simulink model "MultipleAccessTechniques"  (R2019a)
settings: Solver=VariableStepAuto  StartTime=0.0  StopTime=10  RelTol=1e-3
libraries: commdigbbndpm3 x2, commchan3 x1, commrandsrc3 x1, commsink2 x1, commfilt2 x1, commseqgen3 x1, commutil2 x1
settings Model: Creator=se305  LastModifiedBy=se305

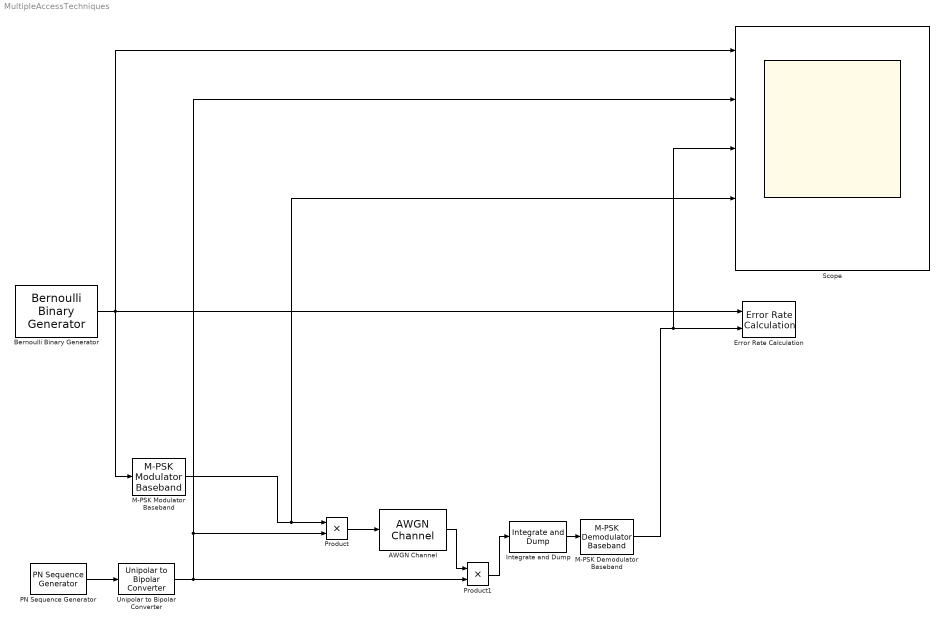
== system MultipleAccessTechniques ==
  AWGN Channel : commchan3/AWGN Channel  InputProcessing=Columns as channels (frame based)  seed=67  noiseMode="Signal to noise ratio  (Eb/No)"  EbNodB=EbNo  EsNodB=10  SNRdB=10  bitsPerSym=1  Ps=1  Tsym=1*(0.001/15)  variance=1
      settings: SourceProductName=Communications Toolbox
  Bernoulli Binary Generator : commrandsrc3/Bernoulli Binary Generator  ProbabilityOfZero=0.5  SeedSource=Auto  Seed=0  SampleTime=0.001  SamplesPerFrame=1  OutputDataType=double  SimulateUsing=Interpreted execution
      settings: SourceProductName=Communications Toolbox
  Error Rate Calculation : commsink2/Error Rate Calculation  N=0  st_delay=0  cp_mode=Entire frame  subframe=[]  PMode=Workspace  WsName=ErrorVec  RsMode2=off  stop=off  numErr=100  maxBits=1e6
      settings: SourceProductName=Communications Toolbox
  Integrate and Dump : commfilt2/Integrate and Dump  obssamples=15  offsetsamples=0  nodump=on  roundingMode=Floor  overflowMode=off  outputDataTypeStr=Inherit: Same as accumulator  outputLastDataTypeStr=Inherit: Same as accumulator
      settings: SourceProductName=Communications Toolbox
  M-PSK Demodulator Baseband : commdigbbndpm3/M-PSK Demodulator Baseband  M=2  OutType=Bit  DecType=Hard decision  VarSource=Dialog  Variance=1  Dec=Binary  Mapping=[0:7]  Ph=0  outDtype1=Inherit via internal rule  outDtype2=Inherit via internal rule  derotateFactorWordLen=16  derotateFactorDataTypeStr=Inherit: Same word length as input  derotateFactorLastDataTypeStr=Inherit: Same word length as input
      settings: SourceProductName=Communications Toolbox
  M-PSK Modulator Baseband : commdigbbndpm3/M-PSK Modulator Baseband  M=2  InType=Bit  Enc=Binary  Mapping=[0:7]  Ph=0  outDtype=double  outWordLen=16  outUDDataType=sfix(16)  outFracLenMode=Best precision  outFracLen=15  outDataTypeStr=double  outLastDataTypeStr=double
      settings: SourceProductName=Communications Toolbox
  PN Sequence Generator : commseqgen3/PN Sequence Generator  poly=[4 3 0]  ini_sta=[0 0 0 1]  outBitMaskSource=Dialog parameter  shift=0  outVarSiz=off  maxOutSizeMode=Dialog parameter  maxOutSize=[10 1]  Ts=0.001/15  sampPerFrame=1  reset=off  bitPackedOutputs=off  outDataType=double  numPackedBits=8  bitPackDataSigned=off  bitPackedOutDType=double
      settings: SourceProductName=Communications Toolbox
  Product : Product
  Product1 : Product
  Scope : Scope  NumInputPorts=5
  Unipolar to Bipolar Converter : commutil2/Unipolar to Bipolar Converter  M=2  polarity=Positive  dataType=Inherit via internal rule
      settings: SourceProductName=Communications Toolbox
  wires:
  M-PSK Demodulator Baseband/1 -> Scope/3, Error Rate Calculation/2
  AWGN Channel/1 -> Product1/1
  PN Sequence Generator/1 -> Unipolar to Bipolar Converter/1
  Product1/1 -> Integrate and Dump/1
  Integrate and Dump/1 -> M-PSK Demodulator Baseband/1
  Product/1 -> AWGN Channel/1
  M-PSK Modulator Baseband/1 -> Scope/4, Product/1
  Bernoulli Binary Generator/1 -> M-PSK Modulator Baseband/1, Scope/1, Error Rate Calculation/1
  Unipolar to Bipolar Converter/1 -> Scope/2, Product/2, Product1/2
